simulink subsystem "ApplianceModel"  (R2023b)
settings: Solver=VariableStepAuto  StartTime=0.0  StopTime=10.0  RelTol=1e-3
model mask{R=0, MinValue=1e-20}
  mask prompts: R "Resistance [ Ω ]"
libraries: fl_lib x3, nesl_utility x2, ee_lib x1
settings Model: Creator=morten  LastModifiedBy=morten

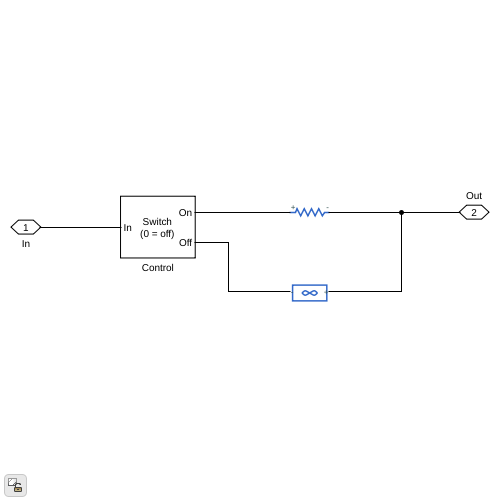
[thumbnail: Simulink's stored preview of the top-level diagram]
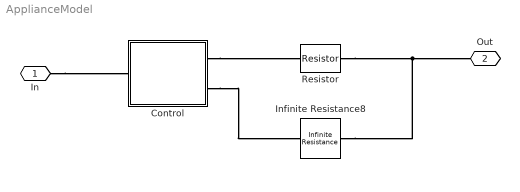
== system ApplianceModel ==
  Control : Subsystem  mask(Switch on){OnBool=R}
      mask prompts: OnBool "On"
      mask help: Connects to OnSignal when the switch is on. Otherwise connects to OffSignal.
      mask Display:
      | on_str = get_param(gcb, 'OnBool');
      | on = strcmp(on_str,'on');
      | 
      | disp("Switch\n(0 = off)")
      | 
      | port_label('lconn', 1, 'In');
      | port_label('rconn', 1, 'On');
      | port_label('rconn', 2, 'Off');
  Infinite Resistance8 : fl_lib/Electrical/Electrical Elements/Infinite Resistance  v_specify=off  v_priority=None  v=0 V  v_nominal_specify=off  v_nominal_unit=V  v_nominal_value=1
      settings: InternalSimscapePortConfiguration="{\"Bottom\":[],\"Left\":[{\"id\":\"p\",\"label\":\"+\",\"type\":\"foundation.electrical.electrical\"}],\"Right\":[{\"id\":\"n\",\"label\":\"-\",\"type\":\"foundation.electrical.electrical\"}],\"Top\":[]}"
  Resistor : ee_lib/Passive/Resistor  R=max(R, MinValue) Ohm  enable_R_tol=ee.enum.toleranceApplication.none  R_tol=5  tol_distribution=ee.enum.toleranceDistribution.uniform  nSigma=4  enable_operating_limits=ee.enum.enable.no  operating_limit_action=ee.enum.passive.reportOpLim.warn  power_rating=1 W  max_working_voltage=100 V  enable_faults=ee.enum.enable.no  fault_action=simscape.enum.assert.action.none  R_faulted=inf Ohm  fault_trigger=ee.enum.faults.faultTrigger.temporal  t_fault=1 s  max_permissible_current=1 A  t_fail_on_current=1 s  noise_mode=ee.enum.sources.noise.Disabled  Tdevice=25 degC  sample_time=1e-3 s  repeatability=ee.enum.ic.repeatability.notRepeatable  user_seed=0  auto_seed=4112460543  faulted_specify=off  faulted_priority=None  faulted=0  power_derating_T1=70 degC  power_derating_T2=155 degC  operating_temperature_range_vec=[-50, 150] degC  alpha=3.93e-3 1/K  Tmeas=25 degC  thermal_mass=100 J/K  temperature_specify=off  temperature_priority=High  temperature=298.15 K  temperature_nominal_specify=off  temperature_nominal_unit=K  temperature_nominal_value=1
  In : PMIOPort  Side=Left
  Out : PMIOPort  Port=2  Side=Right
  connections:
  Infinite Resistance8/LConn1 -- Resistor/RConn1 -- Out/RConn1
  Control/RConn2 -- Infinite Resistance8/RConn1
  In/RConn1 -- Control/LConn1
  Control/RConn1 -- Resistor/LConn1

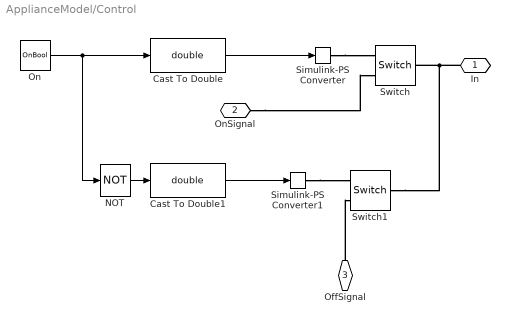
== system ApplianceModel/Control ==
  Cast To Double : DataTypeConversion  OutDataTypeStr=double  SaturateOnIntegerOverflow=off  RndMeth=Floor
  Cast To Double1 : DataTypeConversion  OutDataTypeStr=double  SaturateOnIntegerOverflow=off  RndMeth=Floor
  NOT : Logic  Operator=NOT  IconShape=distinctive  AllPortsSameDT=off  OutDataTypeStr=boolean
  On : Constant  Value=OnBool  OutDataTypeStr=boolean
  Simulink-PS Converter : nesl_utility/Simulink-PS Converter  PhysicalDomain=network_engine_domain  SubClassName=ps_input  LeftPortType=input  RightPortType=output  PseudoPeriodic=off  Frequencies=[]  NoiseDistribution=none  NoiseParameters=[]  Unit=1  AffineConversion=off  FilteringAndDerivatives=provide  SimscapeFilterOrder=1  InputFilterTimeConstant=0.001  UdotUserProvided=0
  Simulink-PS Converter1 : nesl_utility/Simulink-PS Converter  PhysicalDomain=network_engine_domain  SubClassName=ps_input  LeftPortType=input  RightPortType=output  PseudoPeriodic=off  Frequencies=[]  NoiseDistribution=none  NoiseParameters=[]  Unit=1  AffineConversion=off  FilteringAndDerivatives=provide  SimscapeFilterOrder=1  InputFilterTimeConstant=0.001  UdotUserProvided=0
  Switch : fl_lib/Electrical/Electrical Elements/Switch  R_closed=1e-18 Ohm  G_open=1e-18 1/Ohm  Threshold=0.5  i_specify=off  i_priority=None  i=0 A  i_nominal_specify=off  i_nominal_unit=A  i_nominal_value=1  v_specify=off  v_priority=None  v=0 V  v_nominal_specify=off  v_nominal_unit=V  v_nominal_value=1
  Switch1 : fl_lib/Electrical/Electrical Elements/Switch  R_closed=1e-18 Ohm  G_open=1e-18 1/Ohm  Threshold=0.5  i_specify=off  i_priority=None  i=0 A  i_nominal_specify=off  i_nominal_unit=A  i_nominal_value=1  v_specify=off  v_priority=None  v=0 V  v_nominal_specify=off  v_nominal_unit=V  v_nominal_value=1
  In : PMIOPort  Side=Left
  OnSignal : PMIOPort  Port=2  Side=Right
  OffSignal : PMIOPort  Port=3  Side=Right
  wires:
  NOT/1 -> Cast To Double1/1
  On/1 -> NOT/1, Cast To Double/1
  Cast To Double1/1 -> Simulink-PS Converter1/1
  Cast To Double/1 -> Simulink-PS Converter/1
  connections:
  OffSignal/RConn1 -- Switch1/RConn2
  Simulink-PS Converter1/RConn1 -- Switch1/RConn1
  Switch1/LConn1 -- Switch/LConn1 -- In/RConn1
  OnSignal/RConn1 -- Switch/RConn2
  Simulink-PS Converter/RConn1 -- Switch/RConn1
